simulink model "controlMirror"  (R2013b)
settings: Solver=FixedStepDiscrete  SolverMode=SingleTasking  StartTime=0.0  StopTime=20  FixedStep=Ts  RelTol=1e-3
undefined symbols (not defined in the file): transferMatrix, Ts
libraries: rtai_devices x8, simulink x1
settings Model: ExtModeAutoUpdateStatusClock=off  Creator=bucher  LastModifiedBy=rtai-ao
settings DataIOCC: SignalLoggingSaveFormat=ModelDataLogs  SignalLoggingName=sigsOut
settings OptimizationCC: EfficientFloat2IntCast=on  SimCompilerOptimization=On
settings DebuggingCC: SaveWithParameterizedLinksMsg=none  SignalResolutionControl=TryResolveAllWithWarning  SolverPrmCheckMsg=none  MultiTaskDSMMsg=warning  MultiTaskCondExecSysMsg=none
settings HardwareCC: ProdBitPerLong=64  ProdBitPerPointer=64  ProdIntDivRoundTo=Zero  ProdEndianess=LittleEndian  ProdWordSize=64  ProdHWDeviceType=Intel->x86-64  TargetBitPerLong=64  TargetBitPerPointer=64  TargetLongLongMode=on  TargetIntDivRoundTo=Zero  TargetEndianess=LittleEndian  TargetWordSize=64  TargetHWDeviceType=MATLAB Host
settings ModelReferenceCC: UpdateModelReferenceTargets=Force
settings SFSimCC: SFSimEnableDebug=off  SFSimEcho=off  SimCtrlC=off  SimIntegrity=off  SimBuildMode=sf_nonincremental_build
settings RTWCC: SystemTargetFile=rtai.tlc  TemplateMakefile=rtai.tmf  Description=Linux RTAI Real-Time Target  RetainRTWFile=on  ProcessScript=rtai_make_rtw_hook  IncludeERTFirstTime=on
settings CodeAppCC: SimulinkBlockComments=off
settings STFCustomTargetCC: ModelReferenceCompliant=off  GeneratePreprocessorConditionals=Disable all  MATLABClassNameForMDSCustomization=Simulink.SoftwareTarget.TargetSpecificTriggerConfigurationBase  SystemTargetFile=rtai.tlc

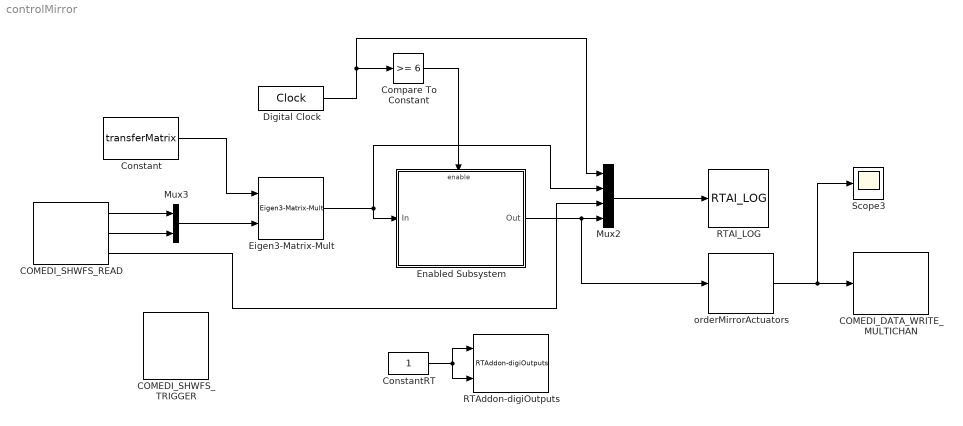
== system controlMirror ==
  COMEDI_DATA_WRITE_MULTICHAN : rtai_devices/COMEDI_DATA_WRITE_MULTICHAN  dev=comedi0  chan=0  nb_chan=64  range=0  aref=ground
  COMEDI_SHWFS_READ : rtai_devices/COMEDI_SHWFS_READ  dev=comedi0  memSize=196  dt=Ts  rePos=on  resolution=on  refEna=on  binaryVector=refBinaryVector  refXVect=refXVector  refYVect=refYVector
  COMEDI_SHWFS_TRIGGER : rtai_devices/COMEDI_SHWFS_TRIGGER  dev=comedi0  dt=Ts_shwfs
  Compare To Constant : simulink/Logic and Bit Operations/Compare To Constant  relop=>=  const=6  OutDataTypeStr=boolean
  Constant : Constant  RequirementInfo={'linktype_rmi_matlab' 'sfun_comedi_shwfs_read' '@' 'true' '} #endif' '' } %GIDa_0b0c33a1_bbc4_46fb_a9cb_4c86aa3513bc  Value=transferMatrix  VectorParams1D=off  SampleTime=Ts
  ConstantRT : Constant  RequirementInfo={'linktype_rmi_matlab' 'sfun_comedi_shwfs_read' '@' 'true' '} #endif' '' } %GIDa_4f86272b_00ac_40df_883d_57bf03db1307  OutDataTypeStr=int32  SampleTime=Ts
  Digital Clock : DigitalClock  SampleTime=Ts
  Eigen3-Matrix-Mult : rtai_devices/Eigen3-Matrix-Mult
  Enabled Subsystem : Subsystem  TreatAsAtomicUnit=on
  Mux2 : Mux
  Mux3 : Mux  Inputs=2
  RTAI_LOG : rtai_devices/RTAI_LOG  dt=Ts
  RTAddon-digiOutputs : rtai_devices/RTAddon-digiOutputs  dev=comedi0  select1=Input signal 1  select2=Input signal 2
  Scope3 : Scope
      settings: SaveName=ScopeData4
  orderMirrorActuators : rtai_devices/orderMirrorActuators  mat=[43,45,11,12, 4, 6,46,40,44,34,32,42,14,21,26,18,19, 1, 5, 3,49,47,38,41]  cntOutput=64  defaultVolt=5.0
  wires:
  Digital Clock/1 -> Mux2/1, Compare To Constant/1
  Compare To Constant/1 -> Enabled Subsystem/Enable
  Mux2/1 -> RTAI_LOG/1
  COMEDI_SHWFS_READ/3 -> Mux2/3
  Constant/1 -> Eigen3-Matrix-Mult/1
  Mux3/1 -> Eigen3-Matrix-Mult/2
  COMEDI_SHWFS_READ/2 -> Mux3/2
  COMEDI_SHWFS_READ/1 -> Mux3/1
  Eigen3-Matrix-Mult/1 -> Mux2/2, Enabled Subsystem/1(In)
  orderMirrorActuators/1 -> COMEDI_DATA_WRITE_MULTICHAN/1, Scope3/1
  ConstantRT/1 -> RTAddon-digiOutputs/1, RTAddon-digiOutputs/2
  Enabled Subsystem/1(Out) -> orderMirrorActuators/1, Mux2/4

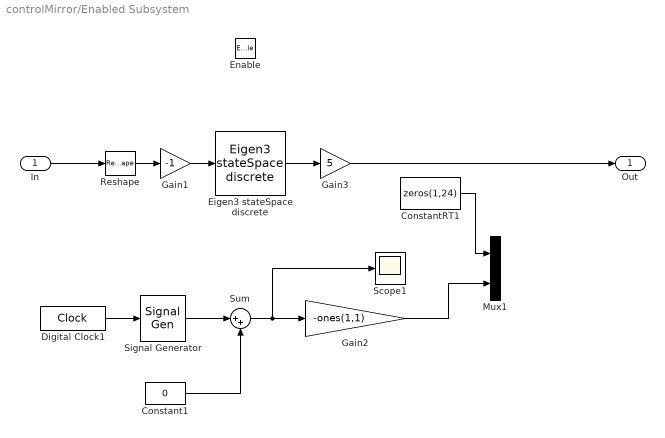
== system controlMirror/Enabled Subsystem ==
  In : Inport
  Enable : EnablePort  StatesWhenEnabling=reset
  Constant1 : Constant  RequirementInfo={'linktype_rmi_matlab' 'sfun_comedi_shwfs_read' '@' 'true' '} #endif' '' } %GIDa_e89d3933_ab72_401f_8c5e_5d2fc43aabc8  Value=0  SampleTime=Ts
  ConstantRT1 : Constant  RequirementInfo={'linktype_rmi_matlab' 'sfun_comedi_shwfs_read' '@' 'true' '} #endif' '' } %GIDa_8adcaf54_f641_4ce2_8bc4_384b8ee0e8fe  Value=zeros(1,24)  OutDataTypeStr=double  SampleTime=Ts
  Digital Clock1 : DigitalClock  SampleTime=Ts
  Eigen3 stateSpace discrete : rtai_devices/Eigen3 stateSpace discrete  matrixA=K1d.A  matrixB=K1d.B  matrixC=K1d.C  matrixD=K1d.D  x0=vect_x0  sampleTime=Ts
  Gain1 : Gain  Gain=-1  OutDataTypeStr=double  SaturateOnIntegerOverflow=on  ParamDataTypeStr=Inherit: Same as input
  Gain2 : Gain  Gain=-ones(1,1)  OutDataTypeStr=double  SaturateOnIntegerOverflow=on  ParamDataTypeStr=Inherit: Same as input
  Gain3 : Gain  Gain=5  OutDataTypeStr=double  SaturateOnIntegerOverflow=on  ParamDataTypeStr=Inherit: Same as input
  Mux1 : Mux  Inputs=2
  Reshape : Reshape
  Scope1 : Scope
  Signal Generator : SignalGenerator  WaveForm=square  TimeSource=Use external signal  Amplitude=5  Frequency=0.002
  Sum : Sum  Inputs=|++
  Out : Outport
  wires:
  In/1 -> Reshape/1
  Reshape/1 -> Gain1/1
  Gain1/1 -> Eigen3 stateSpace discrete/1
  Eigen3 stateSpace discrete/1 -> Gain3/1
  Signal Generator/1 -> Sum/1
  Sum/1 -> Scope1/1, Gain2/1
  Constant1/1 -> Sum/2
  Digital Clock1/1 -> Signal Generator/1
  ConstantRT1/1 -> Mux1/1
  Gain2/1 -> Mux1/2
  Gain3/1 -> Out/1
